simulink model "test_sim"  (R2022b)
settings: Solver=ode4  StartTime=0.0  StopTime=30.0  FixedStep=0.001  RelTol=1e-3
values from neighbouring files (symbols this model uses):
  a = 10    [paraset.m]
  b = 4    [paraset.m]
  Kd = 0    [paraset.m]
  Ki = 0.9    [paraset.m]
  Kp = 0.5    [paraset.m]
settings Model: Creator=user  LastModifiedBy=user
settings DataIOCC: ReturnWorkspaceOutputs=off

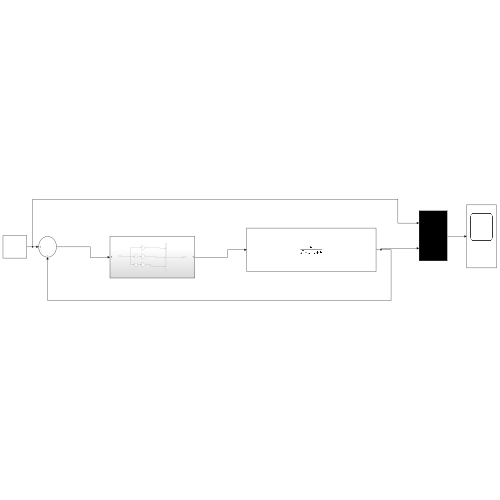
[thumbnail: Simulink's stored preview of the top-level diagram]
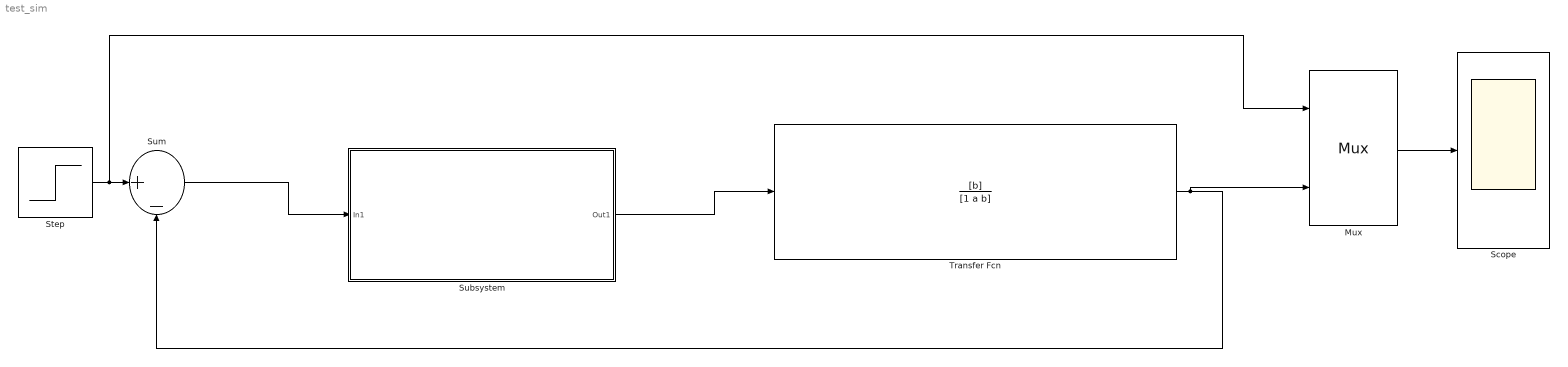
== system test_sim ==
  Mux : Mux  Inputs=2
  Scope : Scope
  Step : Step  SampleTime=0
  Subsystem : Subsystem
  Sum : Sum  Inputs=|+-
  Transfer Fcn : TransferFcn  Numerator=[b]  Denominator=[1 a b]
  wires:
  Transfer Fcn/1 -> Mux/2, Sum/2
  Step/1 -> Mux/1, Sum/1
  Mux/1 -> Scope/1
  Sum/1 -> Subsystem/1(In1)
  Subsystem/1(Out1) -> Transfer Fcn/1

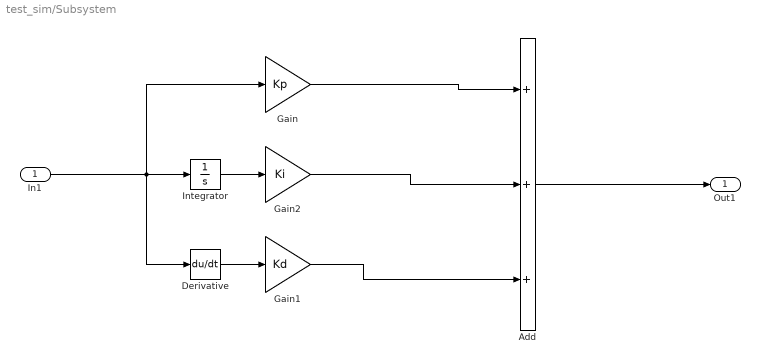
== system test_sim/Subsystem ==
  In1 : Inport
  Add : Sum  Inputs=+++
  Derivative : Derivative
  Gain : Gain  Gain=Kp
  Gain1 : Gain  Gain=Kd
  Gain2 : Gain  Gain=Ki
  Integrator : Integrator
  Out1 : Outport
  wires:
  Derivative/1 -> Gain1/1
  In1/1 -> Gain/1, Derivative/1, Integrator/1
  Integrator/1 -> Gain2/1
  Add/1 -> Out1/1
  Gain2/1 -> Add/2
  Gain/1 -> Add/1
  Gain1/1 -> Add/3
